simulink model "trial_2016"  (R2016b)
settings: Solver=FixedStepDiscrete  StartTime=1  StopTime=2945  FixedStep=1  RelTol=1e-3
values from neighbouring files (symbols this model uses):
  param_init_speed = 0    [go_2016.m]
  param_N = 15    [go_2016.m]
  param_R = 0.001    [go_2016.m]
  param_ref_control = zeros(1,param_traj_len)    [go_2016.m]
  param_ref_speed = Speed(2,:) ./ 3.6    [go_2016.m]
  param_T = 1    [go_2016.m]
undefined symbols (not defined in the file or in its folder): grade
settings Model: Creator=mbatu  LastModifiedBy=mbatu

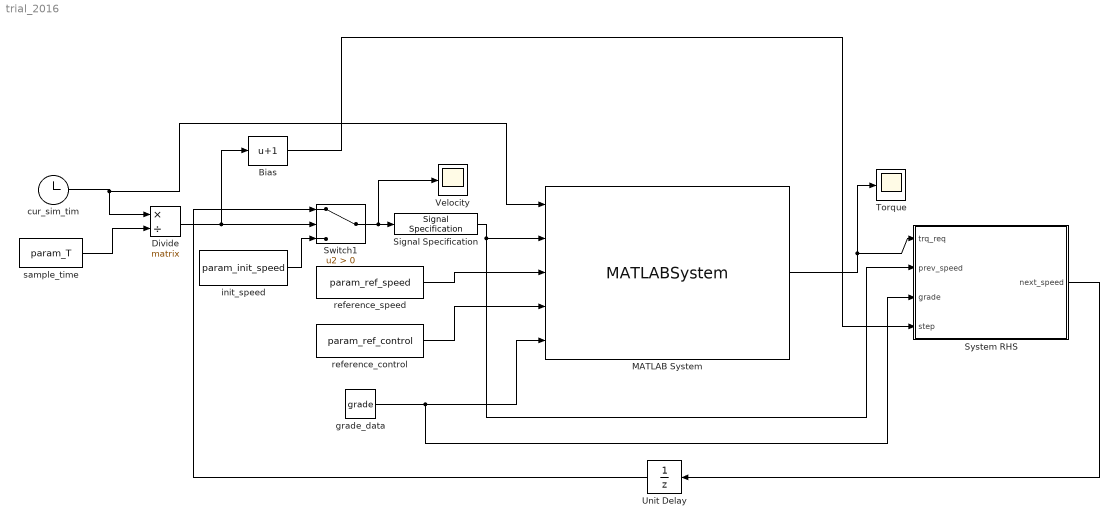
== system trial_2016 ==
  Bias : Bias  Bias=1
  Divide : Product  Inputs=*/  Multiplication=Matrix(*)
  MATLAB System : MATLABSystem  System=MPC_Controller_v2_2016  T=param_T  N=param_N  Q=param_Q  R=param_R  Fbrake=param_Fbrake  Trajlen=param_traj_len  SimulateUsing=Interpreted execution
      mask Type: MPC_Controller_v2_2016
      mask Display:
      | disp('MPC_Controller_v2_2016');
      | port_label('input',1,'cur_sim_tim');
      | port_label('input',2,'cur_speed');
      | port_label('input',3,'ref_speed');
      | port_label('input',4,'ref_control');
      | port_label('input',5,'grade');
      | port_label('output',1,'trq_req');
  Signal Specification : SignalSpecification  OutDataTypeStr=double  Dimensions=[1,1]
  Switch1 : Switch  Criteria=u2 > Threshold
  System RHS : MATLAB Function  TreatAsAtomicUnit=on
  Torque : Scope
  Unit Delay : UnitDelay  SampleTime=-1
  Velocity : Scope
  cur_sim_tim : Clock
  grade_data : Constant  Value=grade
  init_speed : Constant  Value=param_init_speed
  reference_control : Constant  Value=param_ref_control
  reference_speed : Constant  Value=param_ref_speed  OutDataTypeStr=double
  sample_time : Constant  Value=param_T
  wires:
  cur_sim_tim/1 -> MATLAB System/1, Divide/1
  sample_time/1 -> Divide/2
  System RHS/1(next_speed) -> Unit Delay/1
  reference_speed/1 -> MATLAB System/3
  reference_control/1 -> MATLAB System/4
  MATLAB System/1 -> Torque/1, System RHS/1(trq_req)
  Divide/1 -> Bias/1, Switch1/2
  init_speed/1 -> Switch1/3
  Unit Delay/1 -> Switch1/1
  Signal Specification/1 -> MATLAB System/2, System RHS/2(prev_speed)
  Switch1/1 -> Velocity/1, Signal Specification/1
  grade_data/1 -> MATLAB System/5, System RHS/3(grade)
  Bias/1 -> System RHS/4(step)

== matlab function trial_2016/System RHS ==
  data: trq_req input; prev_speed input; next_speed output; grade input; step input
function next_speed = fcn(trq_req, prev_speed, grade, step)

T = 1;           %sample time

% Constants for Vehicle Dynamics
Rtire  =  0.354;  % radius of tire(m)
G      =  9.81;   % earth's gravitational constant(m/s2)
mu     =  0.09;   % road friction(N) 
rho    =  1.225;  % density of air as a fluid(kg/m3)
Cd     =  0.55;   % air drag coefficient
A      =  5.1;    % vehicle frontal area(m2)
mss    =  4200;   % vehicle mass(kg)
ng     =  0.85;   % tire-specific constant
Im     =  0.18;   % motor inertia(kg*m2)
Gb     =  18.5;   % total gear ratio
 
% Variables for Vehicle Dynamics                                           
Fbrake    =  0;                             % braking force(N)
Grade     =  grade(uint16(step));           % grade(%)
alpha     =  atan(Grade/100);               % degree of slope(rad)
Faero     =  0.5*rho*A*Cd*(prev_speed^2);   % drag force against vehicle(N)
Frub      =  mu*mss*G;                      % rubbing force against tires(N)
Ftire     =  trq_req*Gb/Rtire;              % driving force(N)

dvdt      =  (Ftire - Frub - Faero - mss*G*sin(alpha) - Fbrake)/(mss + Im*Gb^2/(ng*Rtire^2));
next_speed = prev_speed + dvdt * T;
